simulink model "SimulinkTankregulering"  (R2023a)
settings: Solver=VariableStepAuto  StartTime=0.0  StopTime=200  RelTol=1e-3
values from neighbouring files (symbols this model uses):
  A = 1    [MATLABTankregulering.m]
  h_r = 0.5    [MATLABTankregulering.m]
  k = 1    [MATLABTankregulering.m]
  Ki = 3    [MATLABTankregulering.m]
  Kp = 100    [MATLABTankregulering.m]
  p = 1000    [MATLABTankregulering.m]
  T = T_values(i)    [MATLABTankregulering.m]
settings Model: Creator=augus  LastModifiedBy=augus

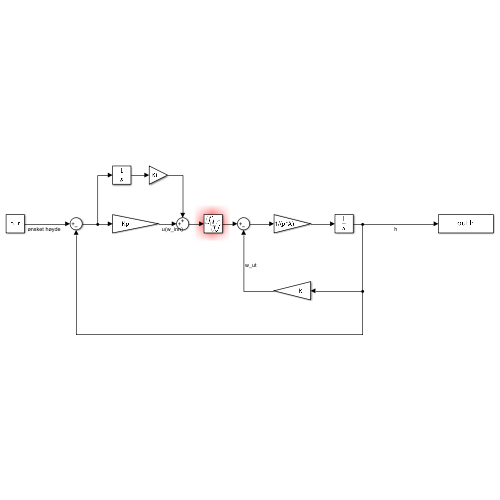
[thumbnail: Simulink's stored preview of the top-level diagram]
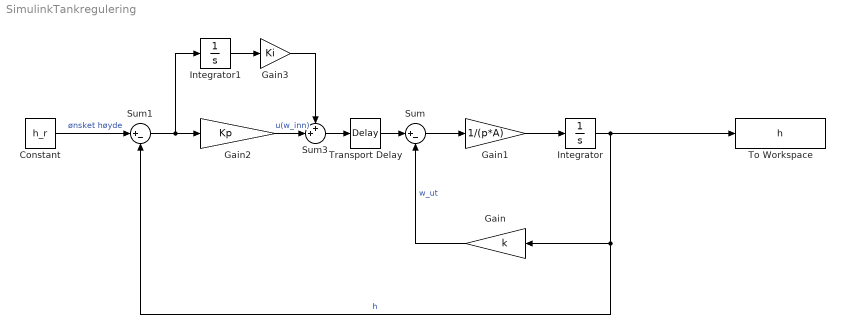
== system SimulinkTankregulering ==
  Constant : Constant  Value=h_r
  Gain : Gain  Gain=k
  Gain1 : Gain  Gain=1/(p*A)
  Gain2 : Gain  Gain=Kp
  Gain3 : Gain  Gain=Ki
  Integrator : Integrator
  Integrator1 : Integrator
  Sum : Sum  Inputs=|+-
  Sum1 : Sum  Inputs=|+-
  Sum3 : Sum  Inputs=++|
  To Workspace : ToWorkspace  VariableName=h  SaveFormat=Timeseries  SampleTime=-1
  Transport Delay : TransportDelay  DelayTime=T
  wires:
  Integrator/1 -> Gain/1, Sum1/2, To Workspace/1  "h"
  Gain/1 -> Sum/2  "w_ut"
  Sum/1 -> Gain1/1
  Gain1/1 -> Integrator/1
  Constant/1 -> Sum1/1  "ønsket høyde"
  Sum1/1 -> Integrator1/1, Gain2/1
  Transport Delay/1 -> Sum/1
  Integrator1/1 -> Gain3/1
  Gain2/1 -> Sum3/2  "u(w_inn)"
  Gain3/1 -> Sum3/1
  Sum3/1 -> Transport Delay/1
